simulink model "IM_Open_loop"  (R2014a)
settings: Solver=FixedStepAuto  StartTime=0.0  StopTime=2  FixedStep=0.0001  RelTol=1e-3
values from neighbouring files (symbols this model uses):
  A1 = [a1 0 a2 0; 0 a1 0 a2; a4 0 a5 0 ; 0 a4 0 a5]    [parametre_IM.m]
  A2 = [0 0 0 a3; 0 0 -a3 0 ; 0 0 0 -1 ; 0 0 1 0]    [parametre_IM.m]
  B = [1/(Ls*sigma) 0; 0 1/(Ls*sigma); 0 0; 0 0]    [parametre_IM.m]
  ClarkConcordia = sqrt(3/2)*[1 -1/2 -1/2; 0 sqrt(3)/2 -sqrt(3)/2; 1/sqrt(2) 1/sqrt(2) 1/sqrt(2)]    [parametre_IM.m]
  ctevf = 240/(2*pi*50)    (= 0.763943726841)    [parametre_IM.m]
  f = 0    [parametre_IM.m]
  J = 0.07    [parametre_IM.m]
  Lr = 0.1568    [parametre_IM.m]
  M = 0.15    [parametre_IM.m]
  p = 2    [parametre_IM.m]
  T = [2/3 -1/3 -1/3; -1/3 2/3 -1/3; -1/3 -1/3 2/3]    [parametre_IM.m]
libraries: simulink x1
settings Model: Creator=TOSHIBA  LastModifiedBy=User
settings DataIOCC: LimitDataPoints=off  SaveFormat=Dataset  ReturnWorkspaceOutputs=on
settings OptimizationCC: LifeSpan=auto  SimCompilerOptimization=off
settings DebuggingCC: MergeDetectMultiDrivingBlocksExec=error  SolverPrmCheckMsg=none  FcnCallInpInsideContextMsg=error  FrameProcessingCompatibilityMsg=error  SFUnexpectedBacktrackingDiag=error  SFNoUnconditionalDefaultTransitionDiag=error
settings HardwareCC: ProdBitPerPointer=64  ProdLargestAtomicFloat=Float  ProdIntDivRoundTo=Zero  ProdEndianess=LittleEndian  ProdWordSize=64  ProdHWDeviceType=Intel->x86-64 (Windows64)
settings ModelReferenceCC: PropagateSignalLabelsOutOfModel=on
settings SFSimCC: SimUseLocalCustomCode=on
settings RTWCC: RTWUseLocalCustomCode=on  RTWCompilerOptimization=off
settings GRTTargetCC: TargetLangStandard=C99 (ISO)  GeneratePreprocessorConditionals=Use local settings

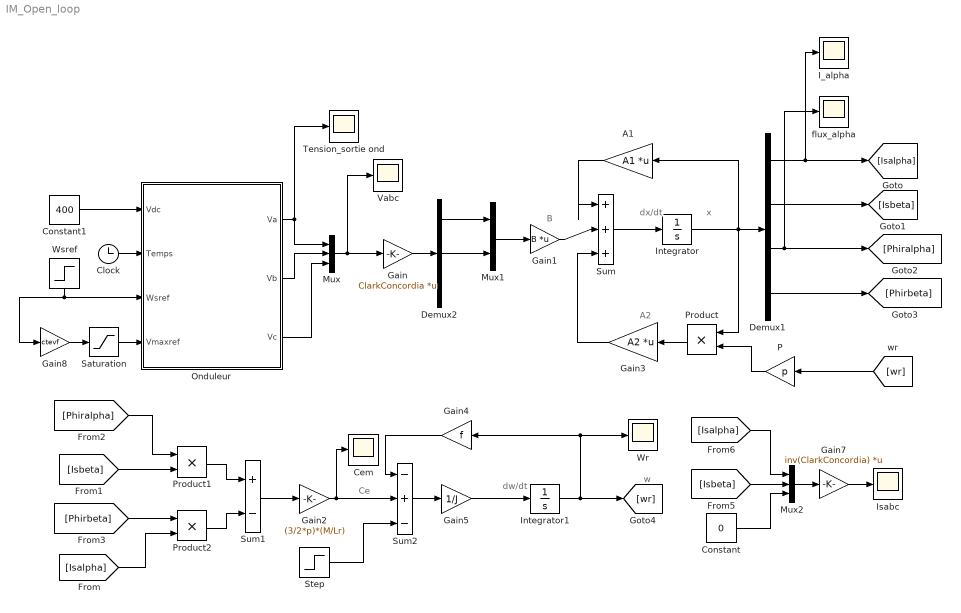
== system IM_Open_loop ==
  note: w
  note: dw/dt
  note: Ce
  note: A2
  note: B
  note: x
  note: dx/dt
  A1 : Gain  Gain=A1  Multiplication=Matrix(K*u)
  Cem : Scope
  Clock : Clock
  Constant : Constant  Value=0
  Constant1 : Constant  Value=400
  Demux1 : Demux
  Demux2 : Demux  Outputs=3
  Gain : Gain  Gain=ClarkConcordia  Multiplication=Matrix(K*u)
  Gain1 : Gain  Gain=B  Multiplication=Matrix(K*u)
  Gain2 : Gain  Gain=(3/2*p)*(M/Lr)
  Gain3 : Gain  Gain=A2  Multiplication=Matrix(K*u)
  Gain4 : Gain  Gain=f
  Gain5 : Gain  Gain=1/J
  Gain7 : Gain  Gain=inv(ClarkConcordia)  Multiplication=Matrix(K*u)
  Gain8 : Gain  Gain=ctevf
  I_alpha : Scope
  Integrator : Integrator
  Integrator1 : Integrator
  Isabc : Scope
  Mux : Mux  Inputs=3
  Mux1 : Mux  Inputs=2
  Mux2 : Mux  Inputs=3
  Onduleur : Subsystem
  P : Gain  Gain=p
  Product : Product
  Product1 : Product
  Product2 : Product
  Saturation : Saturate  UpperLimit=500
  Step : Step  Time=0  After=0  SampleTime=0
  Sum : Sum  Inputs=|+++
  Sum1 : Sum  Inputs=+-
  Sum2 : Sum  Inputs=-+-
  Tension_sortie ond : Scope
  Vabc : Scope
  Wr : Scope
  Wsref : Step  Time=5  Before=2*pi*25  After=2*pi*50  SampleTime=0
  flux_alpha : Scope
  wires:
  Onduleur/1("Va ") -> Tension_sortie ond/1, Mux/1
  Onduleur/2(Vb) -> Mux/2
  Onduleur/3(Vc) -> Mux/3
  Mux/1 -> Vabc/1, Gain/1
  Mux1/1 -> Gain1/1
  Sum/1 -> Integrator/1
  Gain3/1 -> Sum/3
  Integrator/1 -> Demux1/1, A1/1, Product/1
  Product/1 -> Gain3/1
  Demux1/1 -> [Isalpha], I_alpha/1
  Demux1/2 -> [Isbeta]
  Demux1/3 -> flux_alpha/1, [Phiralpha]
  Demux1/4 -> [Phirbeta]
  [Phiralpha] -> Product1/1
  [Isbeta] -> Product1/2
  [Phirbeta] -> Product2/1
  [Isalpha] -> Product2/2
  Product1/1 -> Sum1/1
  Product2/1 -> Sum1/2
  Sum1/1 -> Gain2/1
  Gain2/1 -> Sum2/2, Cem/1
  Sum2/1 -> Gain5/1
  Gain5/1 -> Integrator1/1
  Integrator1/1 -> Gain4/1, Wr/1, [wr]
  [wr] -> P/1
  P/1 -> Product/2
  Gain7/1 -> Isabc/1
  Mux2/1 -> Gain7/1
  [Isalpha] -> Mux2/1
  [Isbeta] -> Mux2/2
  Constant/1 -> Mux2/3
  Demux2/1 -> Mux1/1
  Demux2/2 -> Mux1/2
  Gain/1 -> Demux2/1
  Clock/1 -> Onduleur/2(Temps)
  Wsref/1 -> Onduleur/3(Wsref), Gain8/1
  Constant1/1 -> Onduleur/1(Vdc)
  Gain8/1 -> Saturation/1
  Saturation/1 -> Onduleur/4("Vmaxref ")
  Gain1/1 -> Sum/2
  A1/1 -> Sum/1
  Step/1 -> Sum2/3
  Gain4/1 -> Sum2/1

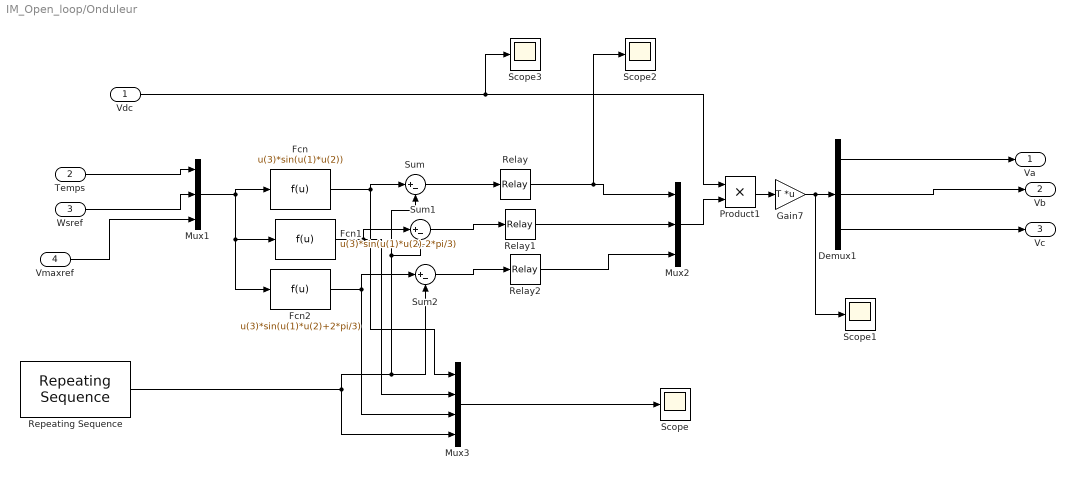
== system IM_Open_loop/Onduleur ==
  Vdc : Inport
  Temps : Inport  Port=2
  Wsref : Inport  Port=3
  "Vmaxref " : Inport  Port=4
  Demux1 : Demux  Outputs=3
  Fcn : Fcn  Expr=u(3)*sin(u(1)*u(2))
  Fcn1 : Fcn  Expr=u(3)*sin(u(1)*u(2)-2*pi/3)
  Fcn2 : Fcn  Expr=u(3)*sin(u(1)*u(2)+2*pi/3)
  Gain7 : Gain  Gain=T  Multiplication=Matrix(K*u)
  Mux1 : Mux  Inputs=3
  Mux2 : Mux  Inputs=3
  Mux3 : Mux
  Product1 : Product
  Relay : Relay  OffOutputValue=-1
  Relay1 : Relay  OffOutputValue=-1
  Relay2 : Relay  OffOutputValue=-1
  Repeating Sequence : simulink/Sources/Repeating Sequence  rep_seq_t=[0 2]  rep_seq_y=[0 2]
  Scope{,1..3} (4 alike) : Scope
  Sum : Sum  Inputs=|+-
  Sum1 : Sum  Inputs=|+-
  Sum2 : Sum  Inputs=|+-
  "Va " : Outport
  Vb : Outport  Port=2
  Vc : Outport  Port=3
  wires:
  Repeating Sequence/1 -> Sum/2, Sum1/2, Sum2/2, Mux3/4
  Mux2/1 -> Product1/2
  Mux1/1 -> Fcn2/1, Fcn1/1, Fcn/1
  Demux1/1 -> "Va "/1
  Relay/1 -> Scope2/1, Mux2/1
  Gain7/1 -> Scope1/1, Demux1/1
  Relay1/1 -> Mux2/2
  Sum/1 -> Relay/1
  Demux1/3 -> Vc/1
  Sum1/1 -> Relay1/1
  Fcn2/1 -> Sum2/1, Mux3/3
  Fcn1/1 -> Mux3/2, Sum1/1
  Fcn/1 -> Mux3/1, Sum/1
  Product1/1 -> Gain7/1
  Relay2/1 -> Mux2/3
  Vdc/1 -> Scope3/1, Product1/1
  Sum2/1 -> Relay2/1
  Wsref/1 -> Mux1/2
  Temps/1 -> Mux1/1
  Demux1/2 -> Vb/1
  Mux3/1 -> Scope/1
  "Vmaxref "/1 -> Mux1/3
